simulink model "HLVRTCalculateV5Sim"  (R2016b)
settings: Solver=VariableStepAuto  StartTime=-1.98  StopTime=1.98  RelTol=1e-3
InitFcn:
  | HLVRTCalculateV5
libraries: powerlib x1
settings Model: Creator=wangxiaofei  LastModifiedBy=wangxiaofei

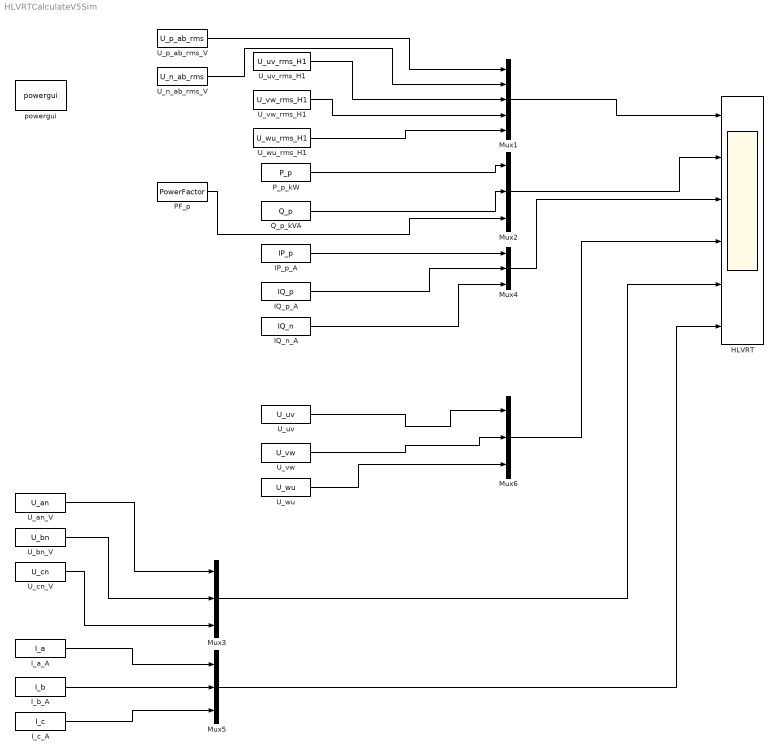
== system HLVRTCalculateV5Sim ==
  HLVRT : Scope  NumInputPorts=6
  IP_p_A : FromWorkspace  VariableName=IP_p  SampleTime=4e-05
  IQ_n_A : FromWorkspace  VariableName=IQ_n  SampleTime=4e-05
  IQ_p_A : FromWorkspace  VariableName=IQ_p  SampleTime=4e-05
  I_a_A : FromWorkspace  VariableName=I_a  SampleTime=4e-05
  I_b_A : FromWorkspace  VariableName=I_b  SampleTime=4e-05
  I_c_A : FromWorkspace  VariableName=I_c  SampleTime=4e-05
  Mux1 : Mux  Inputs=5
  Mux{2..6} (5 alike) : Mux  Inputs=3
  PF_p : FromWorkspace  VariableName=PowerFactor  SampleTime=4e-05
  P_p_kW : FromWorkspace  VariableName=P_p  SampleTime=4e-05
  Q_p_kVA : FromWorkspace  VariableName=Q_p  SampleTime=4e-05
  U_an_V : FromWorkspace  VariableName=U_an  SampleTime=4e-05
  U_bn_V : FromWorkspace  VariableName=U_bn  SampleTime=4e-05
  U_cn_V : FromWorkspace  VariableName=U_cn  SampleTime=4e-05
  U_n_ab_rms_V : FromWorkspace  VariableName=U_n_ab_rms  SampleTime=4e-05
  U_p_ab_rms_V : FromWorkspace  VariableName=U_p_ab_rms  SampleTime=4e-05
  U_uv : FromWorkspace  VariableName=U_uv  SampleTime=4e-05
  U_uv_rms_H1 : FromWorkspace  VariableName=U_uv_rms_H1  SampleTime=4e-05
  U_vw : FromWorkspace  VariableName=U_vw  SampleTime=4e-05
  U_vw_rms_H1 : FromWorkspace  VariableName=U_vw_rms_H1  SampleTime=4e-05
  U_wu : FromWorkspace  VariableName=U_wu  SampleTime=4e-05
  U_wu_rms_H1 : FromWorkspace  VariableName=U_wu_rms_H1  SampleTime=4e-05
  powergui : powerlib/powergui  Priority=1  SimulationMode=Discrete  SolverType=Tustin/Backward Euler (TBE)  SampleTime=1e-06  frequency=60  SPID=off  DisableSnubberDevices=off  DisableRonSwitches=off  DisableVfSwitches=off  SwTol=0  DisplayEquations=off  Interpol=off  ExternalGateDelay=off  methode=off  Ts=10  FunctionMessages=off  echomessages=off  HookPort=off  EnableUseOfTLC=off  x0status=blocks  frequencyindice=60  Pbase=100e6  ErrMax=1e-4  Iterations=50  UnitsV=kV  UnitsW=MW  buscounter=0  RestoreLinks=warning  ResistiveCurrentMeasurement=off  Frange=[0:2:500]  Ylog=off  Xlog=on  ShowGrid=off  save=off  variable=ZData  structure=0  ZoomFFT=off  StartTime=0.0  cycles=1  DisplayStyle=1  fundamental=60  FreqAxis=off  MaxFrequency=1000  frequencyindicesteady=1  RmsSteady=1  display=off
  wires:
  U_an_V/1 -> Mux3/1
  U_bn_V/1 -> Mux3/2
  U_cn_V/1 -> Mux3/3
  I_a_A/1 -> Mux5/1
  I_b_A/1 -> Mux5/2
  I_c_A/1 -> Mux5/3
  U_p_ab_rms_V/1 -> Mux1/1
  U_n_ab_rms_V/1 -> Mux1/2
  P_p_kW/1 -> Mux2/1
  Q_p_kVA/1 -> Mux2/2
  IP_p_A/1 -> Mux4/1
  IQ_p_A/1 -> Mux4/2
  IQ_n_A/1 -> Mux4/3
  Mux1/1 -> HLVRT/1
  Mux2/1 -> HLVRT/2
  Mux4/1 -> HLVRT/3
  Mux5/1 -> HLVRT/6
  Mux3/1 -> HLVRT/5
  U_vw_rms_H1/1 -> Mux1/4
  U_uv_rms_H1/1 -> Mux1/3
  U_wu_rms_H1/1 -> Mux1/5
  Mux6/1 -> HLVRT/4
  U_uv/1 -> Mux6/1
  U_vw/1 -> Mux6/2
  U_wu/1 -> Mux6/3
  PF_p/1 -> Mux2/3
